simulink library "env_estimation_lib"  (R2016b)
settings: Solver=VariableStepAuto  StartTime=0.0  StopTime=10.0  RelTol=1e-3
undefined symbols (not defined in the file): fsw_params
libraries: time_conversion_lib x1, gs_prediction_lib x1, mag_vec_LS_lib x1, sgp4_lib_fsw x1, sun_vector_lib x1, time_coord_rotation_lib x1
settings Model: Creator=taylorreynolds  LastModifiedBy=taylorreynolds

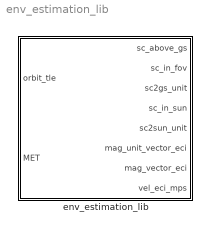
== system env_estimation_lib ==
  env_estimation_lib : Subsystem

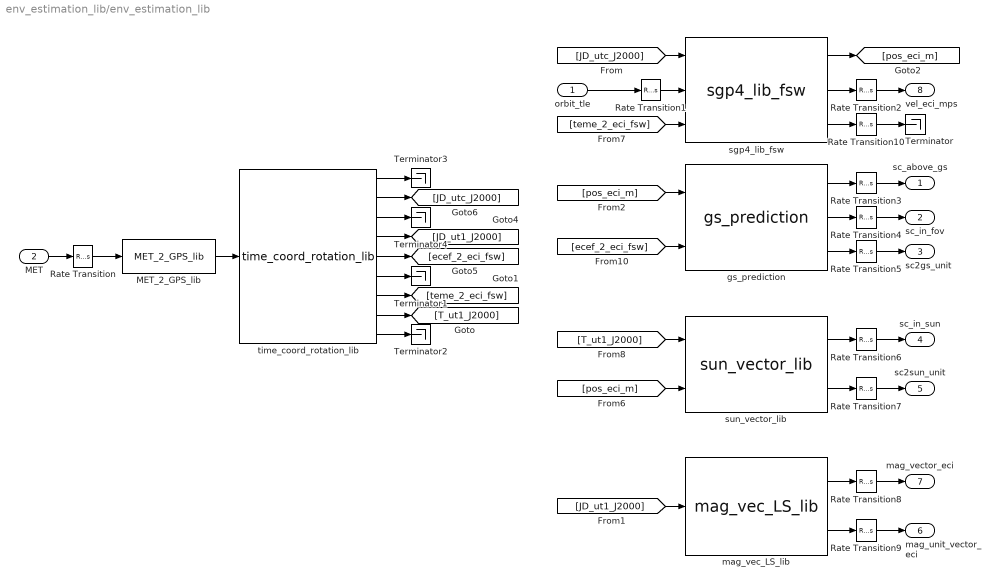
== system env_estimation_lib/env_estimation_lib ==
  orbit_tle : Inport
  MET : Inport  Port=2
  MET_2_GPS_lib : time_conversion_lib/MET_2_GPS_lib
  Rate Transition : RateTransition  X0=fsw_params.sensor_processing.gps.JD_J2000_TT_s  OutPortSampleTime=fsw_params.env_estimation.sample_time_s
  Rate Transition1 : RateTransition  X0=fsw_params.env_estimation.ic.orbit_tle  OutPortSampleTime=fsw_params.env_estimation.sample_time_s
  Rate Transition{2..10} (9 alike) : RateTransition
  Terminator{,1..4} (5 alike) : Terminator
  gs_prediction : gs_prediction_lib/gs_prediction
  mag_vec_LS_lib : mag_vec_LS_lib/mag_vec_LS_lib
  sgp4_lib_fsw : sgp4_lib_fsw/sgp4_lib_fsw
  sun_vector_lib : sun_vector_lib/sun_vector_lib
  time_coord_rotation_lib : time_coord_rotation_lib/time_coord_rotation_lib
  sc_above_gs : Outport
  sc_in_fov : Outport  Port=2
  sc2gs_unit : Outport  Port=3
  sc_in_sun : Outport  Port=4
  sc2sun_unit : Outport  Port=5
  mag_unit_vector_eci : Outport  Port=6
  mag_vector_eci : Outport  Port=7
  vel_eci_mps : Outport  Port=8
  wires:
  mag_vec_LS_lib/2 -> Rate Transition9/1
  mag_vec_LS_lib/1 -> Rate Transition8/1
  sun_vector_lib/2 -> Rate Transition7/1
  [T_ut1_J2000] -> sun_vector_lib/1
  [JD_utc_J2000] -> sgp4_lib_fsw/1
  sun_vector_lib/1 -> Rate Transition6/1
  [pos_eci_m] -> sun_vector_lib/2
  sgp4_lib_fsw/1 -> [pos_eci_m]
  orbit_tle/1 -> Rate Transition1/1
  MET/1 -> Rate Transition/1
  time_coord_rotation_lib/1 -> Terminator3/1
  gs_prediction/1 -> Rate Transition3/1
  gs_prediction/3 -> Rate Transition5/1
  gs_prediction/2 -> Rate Transition4/1
  Rate Transition1/1 -> sgp4_lib_fsw/2
  Rate Transition2/1 -> vel_eci_mps/1
  Rate Transition3/1 -> sc_above_gs/1
  Rate Transition4/1 -> sc_in_fov/1
  Rate Transition5/1 -> sc2gs_unit/1
  Rate Transition6/1 -> sc_in_sun/1
  Rate Transition7/1 -> sc2sun_unit/1
  Rate Transition8/1 -> mag_vector_eci/1
  Rate Transition9/1 -> mag_unit_vector_eci/1
  [ecef_2_eci_fsw] -> gs_prediction/2
  [pos_eci_m] -> gs_prediction/1
  time_coord_rotation_lib/9 -> Terminator2/1
  time_coord_rotation_lib/8 -> [T_ut1_J2000]
  time_coord_rotation_lib/7 -> [teme_2_eci_fsw]
  time_coord_rotation_lib/6 -> Terminator1/1
  time_coord_rotation_lib/5 -> [ecef_2_eci_fsw]
  time_coord_rotation_lib/4 -> [JD_ut1_J2000]
  time_coord_rotation_lib/3 -> Terminator4/1
  time_coord_rotation_lib/2 -> [JD_utc_J2000]
  [teme_2_eci_fsw] -> sgp4_lib_fsw/3
  sgp4_lib_fsw/2 -> Rate Transition2/1
  sgp4_lib_fsw/3 -> Rate Transition10/1
  Rate Transition10/1 -> Terminator/1
  Rate Transition/1 -> MET_2_GPS_lib/1
  MET_2_GPS_lib/1 -> time_coord_rotation_lib/1
  [JD_ut1_J2000] -> mag_vec_LS_lib/1
